simulink model "driving_begginer"  (R2021a)
settings: Solver=VariableStepAuto  StartTime=0.0  StopTime=inf  FixedStep=0.001  RelTol=1e-3
values from neighbouring files (symbols this model uses):
  ref_path1 =     [PATH.mat]
  ref_path2 =     [PATH.mat]
  ref_path3 =     [PATH.mat]
libraries: robotlib x16
settings Model: Creator=harin  LastModifiedBy=harin
settings DataIOCC: ReturnWorkspaceOutputs=off

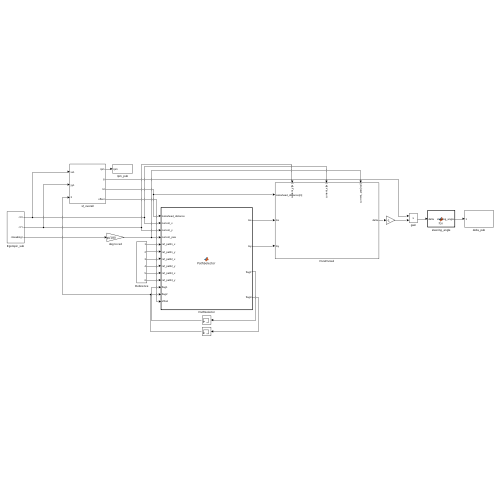
[thumbnail: Simulink's stored preview of the top-level diagram]
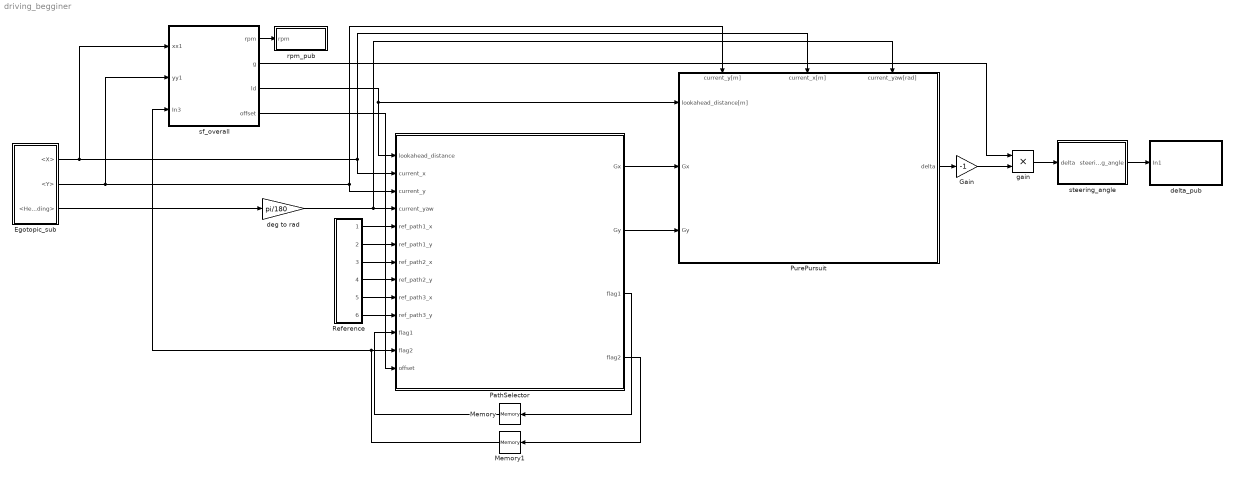
== system driving_begginer ==
  Egotopic_sub : Subsystem
  Gain : Gain  Gain=-1
  Memory : Memory
  Memory1 : Memory
  PathSelector : MATLAB Function  TreatAsAtomicUnit=on
  PurePursuit : Subsystem
      settings: PortSchema="{\"entries\":[{\"content\":{\"sides\":[{\"content\":{\"connectorIds\":[\"In1\",\"In2\",\"In3\"]},\"type\":\"ConnectorPlacement.EquallySpacedRectSide\",\"uuid\":\"edaa732b-c16a-4ee2-a2e3-938fc58760b6\"},{\"content\":{\"connectorIds\":[\"Out1\"],\"side\":\"RIGHT\"},\"type\":\"ConnectorPlacement.EquallySpacedRectSide\",\"uuid\":\"801e571f-7b3b-4885-8003-b37606c63344\"},{\"content\":{\"connectorIds\":[\"In4\",\"In5\",\"In6\"],\"side\":\"TOP\"},\"type\":\"ConnectorPlacement.EquallySpacedRectSide\",\"uuid\":\"9ff8c77f-a710-48d9-b19a-3d1983c753ef\"}]},\"type\":\"ConnectorPlacement.EquallySpacedConnector\",\"uuid\":\"839de6f2-d165-444d-a1b0-1ebd63d9b09d\"}],\"packageUris\":[\"http://schema.mathworks.com/mf0/Connector/R2020b\"],\"version\":\"1.0\"}"
  Reference : Subsystem
  deg to rad : Gain  Gain=pi/180
  delta_pub : Subsystem
  gain : Product
  rpm_pub : Subsystem
  sf_overall : Subsystem
  steering_angle : MATLAB Function  TreatAsAtomicUnit=on
  wires:
  PathSelector/1(Gx) -> PurePursuit/2(Gx)
  Memory/1 -> PathSelector/11("flag1 ")
  PathSelector/2(Gy) -> PurePursuit/3(Gy)
  Memory1/1 -> PathSelector/12("flag2 "), sf_overall/3(In3)
  PathSelector/4(flag2) -> Memory1/1
  PathSelector/3(flag1) -> Memory/1
  deg to rad/1 -> PathSelector/4(current_yaw), PurePursuit/6(current_yaw[rad])
  PurePursuit/1(delta) -> Gain/1
  Gain/1 -> gain/2
  gain/1 -> steering_angle/1(delta)
  steering_angle/1(steering_angle) -> delta_pub/1(In1)
  sf_overall/1(rpm) -> rpm_pub/1(rpm)
  sf_overall/2(g) -> gain/1
  sf_overall/3(ld) -> PathSelector/1(lookahead_distance), PurePursuit/1(lookahead_distance[m])
  sf_overall/4(offset) -> PathSelector/13(offset)
  Egotopic_sub/2(<Y>) -> PurePursuit/4(current_y[m]), PathSelector/3(current_y), sf_overall/2(yy1)
  Egotopic_sub/1(<X>) -> PathSelector/2(current_x), PurePursuit/5(current_x[m]), sf_overall/1(xx1)
  Egotopic_sub/3(<Heading>) -> deg to rad/1
  Reference/1(Out1) -> PathSelector/5(ref_path1_x)
  Reference/2(Out2) -> PathSelector/6(ref_path1_y)
  Reference/3(Out3) -> PathSelector/7(ref_path2_x)
  Reference/4(Out4) -> PathSelector/8(ref_path2_y)
  Reference/5(Out5) -> PathSelector/9(ref_path3_x)
  Reference/6(Out6) -> PathSelector/10(ref_path3_y)

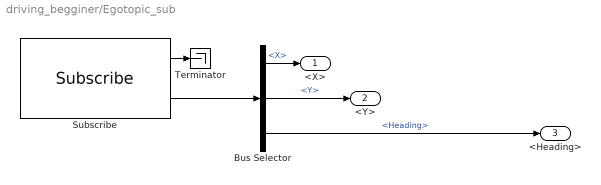
== system driving_begginer/Egotopic_sub ==
  Bus Selector : BusSelector  OutputSignals=Position.X,Position.Y,Heading
  Subscribe : robotlib/Subscribe  topicSource=Select from ROS network  topic=/Ego_topic  messageType=morai_msgs/EgoVehicleStatus  SampleTime=-1  legacyBusStruct=off  messageQueueLength=10
  Terminator : Terminator
  <X> : Outport
  <Y> : Outport  Port=2
  <Heading> : Outport  Port=3
  wires:
  Subscribe/2 -> Bus Selector/1
  Subscribe/1 -> Terminator/1
  Bus Selector/3 -> <Heading>/1  "<Heading>"
  Bus Selector/1 -> <X>/1  "<X>"
  Bus Selector/2 -> <Y>/1  "<Y>"

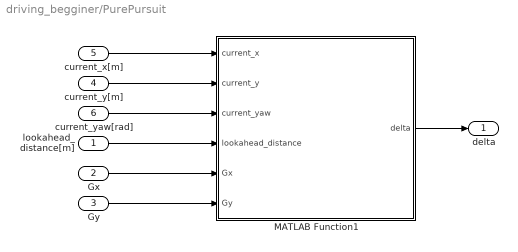
== system driving_begginer/PurePursuit ==
  lookahead_distance[m] : Inport
  Gx : Inport  Port=2
  Gy : Inport  Port=3
  current_y[m] : Inport  Port=4
  current_x[m] : Inport  Port=5
  current_yaw[rad] : Inport  Port=6
  MATLAB Function1 : MATLAB Function  TreatAsAtomicUnit=on
  delta : Outport
  wires:
  current_y[m]/1 -> MATLAB Function1/2(current_y)
  MATLAB Function1/1(delta) -> delta/1
  lookahead_distance[m]/1 -> MATLAB Function1/4(lookahead_distance)
  Gx/1 -> MATLAB Function1/5(Gx)
  Gy/1 -> MATLAB Function1/6(Gy)
  current_yaw[rad]/1 -> MATLAB Function1/3(current_yaw)
  current_x[m]/1 -> MATLAB Function1/1(current_x)

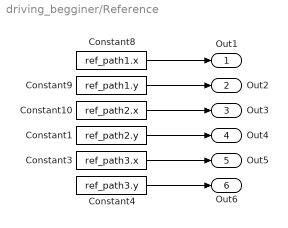
== system driving_begginer/Reference ==
  Constant1 : Constant  Value=ref_path2.y
  Constant10 : Constant  Value=ref_path2.x
  Constant3 : Constant  Value=ref_path3.x
  Constant4 : Constant  Value=ref_path3.y
  Constant8 : Constant  Value=ref_path1.x
  Constant9 : Constant  Value=ref_path1.y
  Out1 : Outport
  Out2 : Outport  Port=2
  Out3 : Outport  Port=3
  Out4 : Outport  Port=4
  Out5 : Outport  Port=5
  Out6 : Outport  Port=6
  wires:
  Constant10/1 -> Out3/1
  Constant9/1 -> Out2/1
  Constant8/1 -> Out1/1
  Constant1/1 -> Out4/1
  Constant4/1 -> Out6/1
  Constant3/1 -> Out5/1

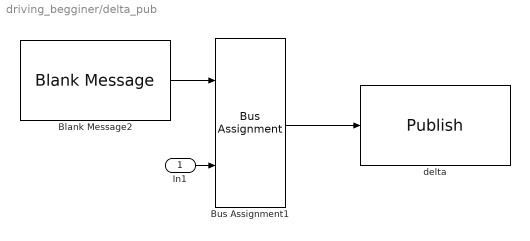
== system driving_begginer/delta_pub ==
  In1 : Inport
  Blank Message2 : robotlib/Blank Message  messageClass=Message  entityType=std_msgs/Float64  messageType=std_msgs/Float64  SampleTime=inf  legacyBusStruct=off
  Bus Assignment1 : BusAssignment  AssignedSignals=Data
  delta : robotlib/Publish  topicSource=Select from ROS network  topic=/commands/servo/position  messageType=std_msgs/Float64  legacyBusStruct=off  messageQueueLength=10
  wires:
  In1/1 -> Bus Assignment1/2
  Blank Message2/1 -> Bus Assignment1/1
  Bus Assignment1/1 -> delta/1

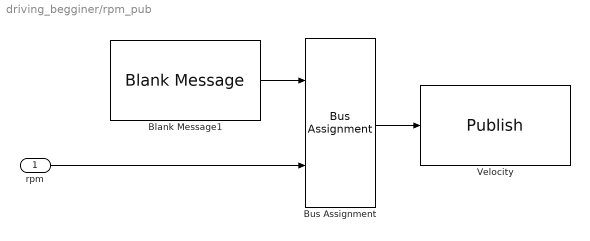
== system driving_begginer/rpm_pub ==
  rpm : Inport
  Blank Message1 : robotlib/Blank Message  messageClass=Message  entityType=std_msgs/Float64  messageType=std_msgs/Float64  SampleTime=inf  legacyBusStruct=off
  Bus Assignment : BusAssignment  AssignedSignals=Data
  Velocity : robotlib/Publish  topicSource=Select from ROS network  topic=/commands/motor/speed  messageType=std_msgs/Float64  legacyBusStruct=off  messageQueueLength=10
  wires:
  rpm/1 -> Bus Assignment/2
  Bus Assignment/1 -> Velocity/1
  Blank Message1/1 -> Bus Assignment/1

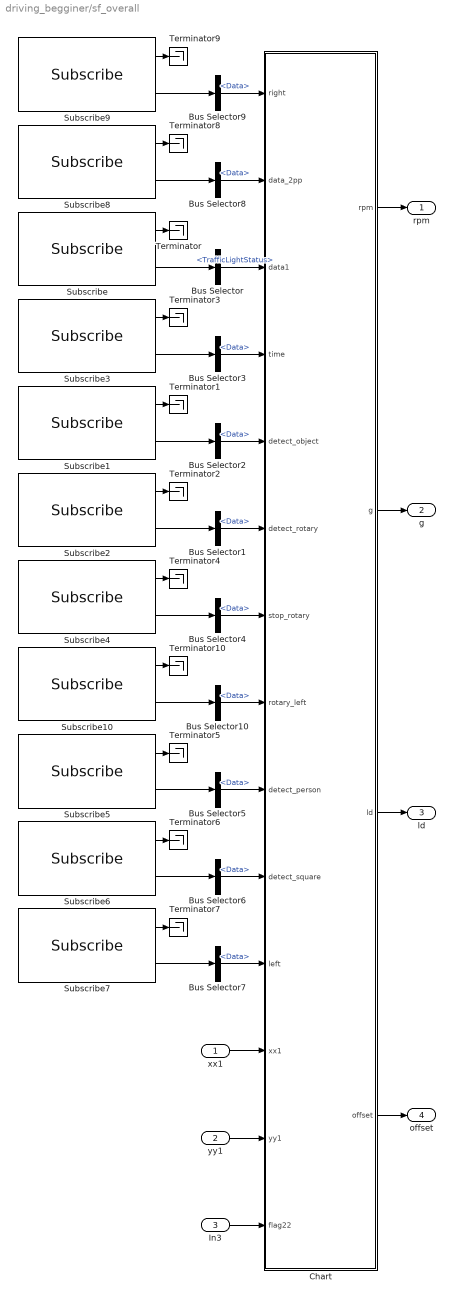
== system driving_begginer/sf_overall ==
  xx1 : Inport
  yy1 : Inport  Port=2
  In3 : Inport  Port=3
  Bus Selector : BusSelector  OutputSignals=TrafficLightStatus
  Bus Selector{1..10} (10 alike) : BusSelector  OutputSignals=Data
  Chart : Stateflow chart  TreatAsAtomicUnit=on
      settings: PortSchema="{\"entries\":[{\"content\":{\"sides\":[{\"content\":{\"connectorIds\":[\"In1\",\"In2\",\"In7\",\"In10\",\"In4\",\"In5\",\"In8\",\"In9\",\"In11\",\"In12\",\"In13\",\"In3\",\"In6\",\"In14\"]},\"type\":\"ConnectorPlacement.EquallySpacedRectSide\",\"uuid\":\"b76d73ed-8faa-4597-b525-d0c269928441\"},{\"content\":{\"connectorIds\":[\"Out1\",\"Out2\",\"Out3\",\"Out4\"],\"side\":\"RIGHT\"},\"type\":\"ConnectorPlacement.EquallySpacedRectSide\",\"uuid\":\"2f5cfc5d-7c35-4e01-a423-3acaa8d67d92\"},{\"content\":{\"connectorIds\":[],\"side\":\"TOP\"},\"type\":\"ConnectorPlacement.EquallySpacedRectSide\",\"uuid\":\"f58eccfd-8b3b-4621-8560-ce1f1d1985bb\"}]},\"type\":\"ConnectorPlacement.EquallySpacedConnector\",\"uuid\":\"8926d43d-d019-4968-9808-4d97be4ca729\"}],\"packageUris\":[\"http://schema.mathworks.com/mf0/Connector/R2020b\"],\"version\":\"1.0\"}"
  Subscribe : robotlib/Subscribe  topicSource=Select from ROS network  topic=/GetTrafficLightStatus  messageType=morai_msgs/GetTrafficLightStatus  SampleTime=-1  legacyBusStruct=off  messageQueueLength=1
  Subscribe1 : robotlib/Subscribe  topicSource=Select from ROS network  topic=/check_object_1  messageType=std_msgs/Int32  SampleTime=-1  legacyBusStruct=off  messageQueueLength=1
  Subscribe10 : robotlib/Subscribe  topicSource=Select from ROS network  topic=/check_rotary_left  messageType=std_msgs/Int32  SampleTime=-1  legacyBusStruct=off  messageQueueLength=1
  Subscribe2 : robotlib/Subscribe  topicSource=Select from ROS network  topic=/check_rotary  messageType=std_msgs/Int32  SampleTime=-1  legacyBusStruct=off  messageQueueLength=1
  Subscribe3 : robotlib/Subscribe  topicSource=Select from ROS network  topic=/timer  messageType=std_msgs/Int32  SampleTime=-1  legacyBusStruct=off  messageQueueLength=1
  Subscribe4 : robotlib/Subscribe  topicSource=Select from ROS network  topic=/stop_rotary  messageType=std_msgs/Int32  SampleTime=-1  legacyBusStruct=off  messageQueueLength=1
  Subscribe5 : robotlib/Subscribe  topicSource=Select from ROS network  topic=/check_person  messageType=std_msgs/Int32  SampleTime=-1  legacyBusStruct=off  messageQueueLength=1
  Subscribe6 : robotlib/Subscribe  topicSource=Select from ROS network  topic=/check_square  messageType=std_msgs/Int32  SampleTime=-1  legacyBusStruct=off  messageQueueLength=1
  Subscribe7 : robotlib/Subscribe  topicSource=Select from ROS network  topic=/check_object_2  messageType=std_msgs/Int32  SampleTime=-1  legacyBusStruct=off  messageQueueLength=1
  Subscribe8 : robotlib/Subscribe  topicSource=Select from ROS network  topic=/check_object_2pp  messageType=std_msgs/Int32  SampleTime=-1  legacyBusStruct=off  messageQueueLength=1
  Subscribe9 : robotlib/Subscribe  topicSource=Select from ROS network  topic=/check_object_3  messageType=std_msgs/Int32  SampleTime=-1  legacyBusStruct=off  messageQueueLength=1
  Terminator{,1..10} (11 alike) : Terminator
  rpm : Outport
  g : Outport  Port=2
  ld : Outport  Port=3
  offset : Outport  Port=4
  wires:
  Chart/1(rpm) -> rpm/1
  yy1/1 -> Chart/6(yy1)
  Chart/3(ld) -> ld/1
  xx1/1 -> Chart/3(xx1)
  Chart/2(g) -> g/1
  Subscribe/2 -> Bus Selector/1
  Bus Selector/1 -> Chart/7(data1)  "<TrafficLightStatus>"
  Subscribe/1 -> Terminator/1
  Subscribe1/1 -> Terminator1/1
  Subscribe2/1 -> Terminator2/1
  Subscribe2/2 -> Bus Selector1/1
  Bus Selector1/1 -> Chart/5(detect_rotary)  "<Data>"
  Subscribe1/2 -> Bus Selector2/1
  Bus Selector2/1 -> Chart/4(detect_object)  "<Data>"
  Subscribe3/1 -> Terminator3/1
  Subscribe3/2 -> Bus Selector3/1
  Bus Selector3/1 -> Chart/10(time)  "<Data>"
  Chart/4(offset) -> offset/1
  Subscribe4/2 -> Bus Selector4/1
  Bus Selector4/1 -> Chart/8(stop_rotary)  "<Data>"
  Subscribe4/1 -> Terminator4/1
  Subscribe5/2 -> Bus Selector5/1
  Bus Selector5/1 -> Chart/11(detect_person)  "<Data>"
  Subscribe5/1 -> Terminator5/1
  Bus Selector6/1 -> Chart/12(detect_square)  "<Data>"
  Subscribe6/2 -> Bus Selector6/1
  Subscribe6/1 -> Terminator6/1
  Subscribe7/1 -> Terminator7/1
  Subscribe7/2 -> Bus Selector7/1
  Bus Selector7/1 -> Chart/13(left)  "<Data>"
  Subscribe8/2 -> Bus Selector8/1
  Bus Selector8/1 -> Chart/2(data_2pp)  "<Data>"
  Subscribe8/1 -> Terminator8/1
  Bus Selector9/1 -> Chart/1(right)  "<Data>"
  Subscribe9/1 -> Terminator9/1
  Subscribe9/2 -> Bus Selector9/1
  In3/1 -> Chart/14(flag22)
  Subscribe10/1 -> Terminator10/1
  Bus Selector10/1 -> Chart/9(rotary_left)  "<Data>"
  Subscribe10/2 -> Bus Selector10/1

== stateflow chart driving_begginer/sf_overall/Chart ==
  state Others1
    du :
    rpm = 0;
    g = 0;
    ld = 0;
  state m3_2
    du :
    rpm = 0;
    ld = 0.8;
    g = 25;
  state m5_2
    du :
    rpm = 10000;
    ld = 1;
    g = 20;
  state m5_3
    du :
    rpm = 0;
    ld = 1;
    g = 20;
  state m4to5
    du :
    rpm = 10000;
    ld = 1;
    g = 20;
  state LeftLight1
    du :
    rpm = 10000;
    ld = 1;
    g = 20;
  state m4
    du :
    rpm = 10000;
    ld = 1;
    g = 20;
  state m4_2
    du :
    rpm = 10000;
    ld = 1;
    g = 20;
  state m3_1
    du :
    rpm = 10000;
    ld = 1;
    g = 20;
  state m5_4
    du :
    rpm = 10000;
    ld = 1;
    g = 20;
  state range_in1
    du :
    offset = 0.42;
  state range_in3
    du :
    offset = 0.42;
  state Others
    du :
    rpm = 0;
    g = 0;
    ld = 0;
  state rotary2
    du :
    rpm = 1500;
    ld = 0.7;
    g = 25;
  state range_in2
    du :
    offset = 0.42;
  state rotary6
    du:
    rpm = 0;
    ld = 0.4;
    g = 17;
  state rotary12
    du:
    rpm = 100;
    ld = 0.5;
    g = 25;
  state m3m3
    du :
    rpm = 10000;
    ld = 1;
    g = 20;
  state rotary10
    du:
    rpm = 1600;
    ld = 0.6;
    g = 30;
  state mission1
    du :
    rpm = 0;
    ld = 0.7;
    g = 10;
  state LeftLight
    du :
    rpm = 10000;
    ld = 1;
    g = 20;
  state m2m3
    du:
    rpm = 10000;
    ld = 0.85;
    g = 19;
  state rotary1
    du:
    rpm = 0;
    ld = 0;
    g = 17;
  state Initial
    du :
    rpm = 10000;
    ld = 0.7;
    g = 10;
  state rotary3
    du:
    rpm =1500;
    ld = 0.7;
    g = 25;
  state mission1_1
    du :
    rpm = 10000;
    ld = 0.7;
    g = 10;
  state m3
    du :
    rpm = 0;
    ld = 0;
    g = 0;
  state m2m33
    du:
    rpm = 10000;
    ld = 0.85;
    g = 19;
  state rotary9
    du:
    rpm = 1600;
    ld = 0.6;
    g = 30;
  state rotary11
    du:
    rpm = 100;
    ld = 0.5;
    g = 25;
  (junction 227) -> Others1 [order 2] : [data1 ~= 33]
  Others1 -> (junction 227) : [data1 == 33]
  m3m3 -> m3_2 : [(yy1<2.5)&&(xx1>6)]
  m3_2 -> (junction 227) : [cal_range(xx1,yy1) == 1]
  (junction 227) -> LeftLight1 [order 1] : [data1 == 33]
  m5_2 -> m5_3 [order 1] : [detect_person==1]{start=time;}
  m5_3 -> m5_2 [order 2] : [detect_person == 0]
  m4to5 -> m5_2 [order 1] : [yy1<-2]
  m5_3 -> m5_4 [order 1] : [(detect_square==0)&&(time-start > 10)]
  m5_2 -> m4to5 [order 2] : [yy1>-2]
  m5_4 -> m5_2 [order 2] : [detect_person==0]
  m4 -> m4to5 : [xx1<0]
  m5_4 -> m5_3 [order 1] : [detect_square==1]
  m4to5 -> m4_2 [order 2] : [yy1>4.2]
  m4_2 -> m4to5 [order 1] : [yy1<4.2]
  LeftLight1 -> m3_1 : [cal_range(xx1,yy1) ~= 1]
  range_in3 -> m4_2 : [(right == 0)]
      | {offset = 0;}
  rotary2 -> m4 [order 1] : [eq_range(yy1,1.9) == 1]
  m4_2 -> range_in1 [order 2] : [detect_object == 1&& yy1> 5.35]
  m3_1 -> rotary6 : [xx1>10.2]{start = time;}
  m4_2 -> range_in2 [order 3] : [left == 1 && flag22 ~= 0 && xx1 > -5]
  range_in1 -> range_in3 : [data_2pp == 1]
  range_in2 -> range_in3 : [data_2pp == 1]
  rotary6 -> rotary2 : [ (detect_rotary == 0) && (rotary_left == 0)  ]
  rotary2 -> rotary10 [order 2] : [(xx1>12)&&(yy1<0)]
  Others -> (junction 141) : [data1 == 33]
  (junction 141) -> Others [order 2] : [data1 ~= 33]
  rotary10 -> rotary2 [order 1] : [yy1>0.9]
  rotary12 -> rotary10 : [stop_rotary == 0]
  rotary10 -> rotary12 [order 2] : [stop_rotary == 1]
  (junction 141) -> LeftLight [order 1] : [data1 == 33]
  LeftLight -> m3m3 : [cal_range(xx1,yy1) ~= 1]
  m3 -> (junction 141)
  mission1_1 -> rotary1 : [xx1<15.4]{start=time;}
  rotary3 -> m2m3 [order 2] : [yy1<-1.68]
  m2m3 -> m2m33 : [yy1<-3.8]
  Initial -> mission1 : [yy1>-2.45]{start = time;}
  (default) -> Initial
  mission1 -> mission1_1 : [time - start == 52 ]
  rotary1 -> rotary3 : [ (detect_rotary == 0) && (rotary_left == 0)  ]
  rotary3 -> rotary9 [order 1] : [(xx1<13.5) && (yy1>0)]
  rotary9 -> rotary3 [order 1] : [yy1<-0.8]
  m2m33 -> m3 : [yy1>-2.45]
  rotary11 -> rotary9 : [stop_rotary == 0]
  rotary9 -> rotary11 [order 2] : [stop_rotary == 1]
  data: x1 function_input; q function_output; ax function_input; x1 function_input; q function_output; y1 function_input; right input; data_2pp input; rpm output; xx1 input; detect_object input; detect_rotary input; yy1 input; g output; ld output; data1 input; stop_rotary input; rotary_left input; time input; start local int32; offset output; detect_person input; detect_square input; left input; flag22 input
  function q  = eq_range(x1,ax):
    | function q  = eq_range(x1,ax)
    | 
    | 
    | aaxp = ax + 0.057; 
    | aaxm = ax - 0.057;
    | if (aaxm < x1) && (x1 < aaxp)
    |     q = 1;
    | else 
    |     q = 0;
    | end
  function q  = cal_range(x1,y1):
    | function q  = cal_range(x1,y1)
    | 
    | % x_range = 5.74:0.01:7.7;
    | % y_range = -2.22:0.01:2.6;
    | 
    | a = x1;
    | b = y1;
    | 
    | if (a > 5.74) && (a < 7.7) && (b < 3) && (b > -2.45)
    |     q = 1;
    | else
    |     q = 0;
    | end

== matlab function driving_begginer/steering_angle ==
  data: delta input; steering_angle output
function steering_angle = fcn(delta)

steering_angle = 0;

if delta > 0
    steering_angle = 0.5+((0.5)/180)*(delta*180/pi);
elseif delta < 0
    steering_angle = 0.5+((0.5)/180)*(delta*180/pi);
elseif delta == 0
    steering_angle = 0.5;
end

== matlab function driving_begginer/PurePursuit/MATLAB Function1 ==
  data: current_x input; delta output; current_y input; current_yaw input; lookahead_distance input; Gx input; Gy input
function delta = fcn(current_x, current_y, current_yaw, lookahead_distance, Gx, Gy)

e_ld = -(Gx-current_x)*sin(current_yaw) + (Gy-current_y)*cos(current_yaw);
sin_alpha = e_ld / lookahead_distance;
L = 0.3;
delta = atan2(2*L*sin_alpha,lookahead_distance);

== matlab function driving_begginer/PathSelector ==
  data: lookahead_distance input; Gx output; current_x input; current_y input; current_yaw input; Gy output; ref_path1_x input; ref_path1_y input; ref_path2_x input; ref_path2_y input; ref_path3_x input; ref_path3_y input; flag1 input; flag2 input; flag1 output; flag2 output; offset input
function [Gx, Gy, flag1, flag2] = PathSelector(lookahead_distance, current_x, current_y, current_yaw, ref_path1_x, ref_path1_y, ref_path2_x, ref_path2_y, ref_path3_x, ref_path3_y, flag1, flag2,offset)
% Select flag
if (current_x > 5.7905) && (current_x < 6.2050) && (current_y > 3.4810) && (current_y < 4.2231)
    flag1 = flag1 + 1;
elseif (current_x > -2.5119) && (current_x < -1.9794) && (current_y > 3.2980) && (current_y < 3.8888)
    flag2 = flag2 + 1;
end

reference_x = ref_path1_x;
reference_y = ref_path1_y;

if (flag1 == 0) && (flag2 == 0)
    reference_x = ref_path1_x;
    reference_y = ref_path1_y;
elseif (flag1 ~= 0) && (flag2 == 0)
    reference_x = ref_path2_x;
    reference_y = ref_path2_y;
    reference_y = reference_y - offset;
elseif (flag1 ~= 0) && (flag2 ~= 0)
    reference_x = ref_path3_x;
    reference_y = ref_path3_y;
    reference_y = reference_y - offset;
end

% Gx,Gy
gx = current_x+lookahead_distance*cos(current_yaw);
gy = current_y+lookahead_distance*sin(current_yaw);
distance = sqrt((gx-reference_x).^2+(gy-reference_y).^2);
[value,index] = min(distance);
Gx = reference_x(index);
Gy = reference_y(index);
end
